simulink model "IEEE123bus_v2019b_Phasor_DPL_ZIPload"  (R2019b)
settings: Solver=VariableStepAuto  StartTime=0.0  StopTime=100  FixedStep=Ts  RelTol=1e-3
InitFcn:
  | a=1; % Loading Factor
  | Ts=0.1;% For Delay Blocks in Voltage Regulator Controls
  | 
  | % Simulation data for the IEEE 123 Node Test Feeder model
  | mi2km = 1.60934;%  miles to km conversion
  | ft2km = 0.0003048; % feet to km conversion
  | ms2F = 1*1e-6/(2*pi*60);% microsiemens to Farads conversion
  | 
  | %% Configuration 1
  | % Series Resitance and Reactance - ohm/mile
  | R_1 = [0.4576 0.1560 0.1535;0.1560 0.4666 0.1580;0.1535 0.1580 0.4615];
  | X_1 = [1.0780 0.5017 0.3849;0.5017 1.0482 0.4236;0.3849 0.4236 1.0651];
  | % charging susceptance - microsiemens/mile
  | B_1 = [5.6765 -1.8319 -0.6982;-1.8319 5.9809 -1.1645;-0.6982 -1.1645 5.3971];
  | 
  | R_1 = R_1/mi2km;
  | L_1 = (X_1/(2*pi*60))/mi2km;
  | C_1 =(B_1*ms2F)/mi2km;
  | 
  | %% Configuration 2 - series reactance - ohm/mile
  | R_2 = [0.4666 0.1580 0.1560;0.1580 0.4615 0.1535;0.1560 0.1535 0.4576];
  | X_2 = [1.0482 0.4236 0.5017;0.4236 1.0651 0.3849;0.5017 0.3849 1.0780];
  | % charging susceptance - microsiemens/mile
  | B_2 = [5.9809 -1.1645 -1.8319;-1.1645 5.3971 -0.6982;-1.8319 -0.6982 5.6765];
  | 
  | R_2 = R_2/mi2km;
  | L_2 = (X_2/(2*pi*60))/mi2km;
  | C_2 =(B_2*ms2F)/mi2km;
  | 
  | %% Configuration 3 - series reactance - ohm/mile
  | R_3 = [0.4615 0.1535 0.1580;0.1535 0.4576 0.1560;0.1580 0.1560 0.4666];
  | X_3 = [1.0651 0.3849 0.4236;0.3849 1.0780 0.5017;0.4236 0.5017 1.0482];
  | % charging susceptance - microsiemens/mile
  | B_3 = [5.3971 -0.6982 -1.1645;-0.6982 5.6765 -1.8319; -1.1645 -1.8319 5.9809];
  | 
  | R_3 = R_3/mi2km;
  | L_3 = (X_3/(2*pi*60))/mi2km;
  | C_3 =(B_3*ms2F)/mi2km;
  | 
  | %% Configuration 4 - series reactance - ohm/mile
  | R_4 = [0.4615 0.1580 0.1535;0.1580 0.4666 0.1560;0.1535 0.1560 0.4576];
  | X_4 = [1.0651 0.4236 0.3849;0.4236 1.0482 0.5017;0.3849 0.5017 1.0780];
  | % charging susceptance - microsiemens/mile
  | B_4 = [5.3971 -1.1645 -0.6982;-1.1645 5.9809 -1.8319;-0.6982 -1.8319 5.6765];
  | 
  | R_4 = R_4/mi2km;
  | L_4 = (X_4/(2*pi*60))/mi2km;
  | C_4 =(B_4*ms2F)/mi2km;
  | 
  | %% Configuration 5 - series reactance - ohm/mile
  | R_5 = [0.4666 0.1560 0.1580;0.1560 0.4576 0.1535;0.1580 0.1535 0.4615];
  | X_5 = [1.0482 0.5017 0.4236;0.5017 1.0780 0.3849;0.4236 0.3849 1.0651];
  | % charging susceptance - microsiemens/mile
  | B_5 = [5.9809 -1.8319 -1.1645;-1.8319 5.6765 -0.6982;-1.1645 -0.6982 5.3971];
  | 
  | R_5 = R_5/mi2km;
  | L_5 = (X_5/(2*pi*60))/mi2km;
  | C_5 =(B_5*ms2F)/mi2km;
  | 
  | %% Configuration 6 - series reactance - ohm/mile
  | ... (+68 lines)
undefined symbols (not defined in the file or in its folder): D1, Delta, find_system, j
libraries: powerlib x886, powerlib_meascontrol x31
(part 12 of 12)

== matlab function IEEE123bus_v2019b_Phasor_DPL_ZIPload/114 Y PQ/Embedded MATLAB Function ==
  data: Iinj output; Vmeas input; LoadType parameter; Vnom parameter; Pnom parameter; Qnom parameter; Vlim parameter
%Single Phase ZIP Load
%Author: Arun Suresh, University of North Carolina, Charlotte
%Iinj=((Pnom+jQnom)/Vmeas)'
function Iinj = InjectedCurrent(Vmeas,LoadType,Vnom,Pnom,Qnom,Vlim)
% Calculate Pl and Ql.
Kz=0;Ki=0;Kp=0;
Vk=(abs(Vmeas)/Vnom);%(Vmeas/Vnom)
switch LoadType  % 1 for Constant Z, 2 for Constant I and 3 for Constant P, 
    case 1
        Kz=1;
    case 2
        if Vk >= Vlim % convert to Constant Z load due to voltage violation
            Ki=1;
        else
            Kz=1;
        end
    case 3
        if Vk >= Vlim % convert to Constant Z load due to voltage violation
           Kp=1;
        else
            Kz=1;
        end          
 
end
Pl=Pnom *((Kz*Vk*Vk)+(Ki*Vk)+(Kp));
Ql=Qnom *((Kz*Vk*Vk)+(Ki*Vk)+(Kp));
% Net Injected Curent.
% j=sqrt(-1);
Iinj = conj((Pl+j*Ql)/Vmeas);

== matlab function IEEE123bus_v2019b_Phasor_DPL_ZIPload/113 Y Z/Embedded MATLAB Function ==
  data: Iinj output; Vmeas input; LoadType parameter; Vnom parameter; Pnom parameter; Qnom parameter; Vlim parameter
%Single Phase ZIP Load
%Author: Arun Suresh, University of North Carolina, Charlotte
%Iinj=((Pnom+jQnom)/Vmeas)'
function Iinj = InjectedCurrent(Vmeas,LoadType,Vnom,Pnom,Qnom,Vlim)
% Calculate Pl and Ql.
Kz=0;Ki=0;Kp=0;
Vk=(abs(Vmeas)/Vnom);%(Vmeas/Vnom)
switch LoadType  % 1 for Constant Z, 2 for Constant I and 3 for Constant P, 
    case 1
        Kz=1;
    case 2
        if Vk >= Vlim % convert to Constant Z load due to voltage violation
            Ki=1;
        else
            Kz=1;
        end
    case 3
        if Vk >= Vlim % convert to Constant Z load due to voltage violation
           Kp=1;
        else
            Kz=1;
        end          
 
end
Pl=Pnom *((Kz*Vk*Vk)+(Ki*Vk)+(Kp));
Ql=Qnom *((Kz*Vk*Vk)+(Ki*Vk)+(Kp));
% Net Injected Curent.
% j=sqrt(-1);
Iinj = conj((Pl+j*Ql)/Vmeas);

== matlab function IEEE123bus_v2019b_Phasor_DPL_ZIPload/112 Y I/Embedded MATLAB Function ==
  data: Iinj output; Vmeas input; LoadType parameter; Vnom parameter; Pnom parameter; Qnom parameter; Vlim parameter
%Single Phase ZIP Load
%Author: Arun Suresh, University of North Carolina, Charlotte
%Iinj=((Pnom+jQnom)/Vmeas)'
function Iinj = InjectedCurrent(Vmeas,LoadType,Vnom,Pnom,Qnom,Vlim)
% Calculate Pl and Ql.
Kz=0;Ki=0;Kp=0;
Vk=(abs(Vmeas)/Vnom);%(Vmeas/Vnom)
switch LoadType  % 1 for Constant Z, 2 for Constant I and 3 for Constant P, 
    case 1
        Kz=1;
    case 2
        if Vk >= Vlim % convert to Constant Z load due to voltage violation
            Ki=1;
        else
            Kz=1;
        end
    case 3
        if Vk >= Vlim % convert to Constant Z load due to voltage violation
           Kp=1;
        else
            Kz=1;
        end          
 
end
Pl=Pnom *((Kz*Vk*Vk)+(Ki*Vk)+(Kp));
Ql=Qnom *((Kz*Vk*Vk)+(Ki*Vk)+(Kp));
% Net Injected Curent.
% j=sqrt(-1);
Iinj = conj((Pl+j*Ql)/Vmeas);

== matlab function IEEE123bus_v2019b_Phasor_DPL_ZIPload/106 Y PQ/Embedded MATLAB Function ==
  data: Iinj output; Vmeas input; LoadType parameter; Vnom parameter; Pnom parameter; Qnom parameter; Vlim parameter
%Single Phase ZIP Load
%Author: Arun Suresh, University of North Carolina, Charlotte
%Iinj=((Pnom+jQnom)/Vmeas)'
function Iinj = InjectedCurrent(Vmeas,LoadType,Vnom,Pnom,Qnom,Vlim)
% Calculate Pl and Ql.
Kz=0;Ki=0;Kp=0;
Vk=(abs(Vmeas)/Vnom);%(Vmeas/Vnom)
switch LoadType  % 1 for Constant Z, 2 for Constant I and 3 for Constant P, 
    case 1
        Kz=1;
    case 2
        if Vk >= Vlim % convert to Constant Z load due to voltage violation
            Ki=1;
        else
            Kz=1;
        end
    case 3
        if Vk >= Vlim % convert to Constant Z load due to voltage violation
           Kp=1;
        else
            Kz=1;
        end          
 
end
Pl=Pnom *((Kz*Vk*Vk)+(Ki*Vk)+(Kp));
Ql=Qnom *((Kz*Vk*Vk)+(Ki*Vk)+(Kp));
% Net Injected Curent.
% j=sqrt(-1);
Iinj = conj((Pl+j*Ql)/Vmeas);

== matlab function IEEE123bus_v2019b_Phasor_DPL_ZIPload/107 Y PQ/Embedded MATLAB Function ==
  data: Iinj output; Vmeas input; LoadType parameter; Vnom parameter; Pnom parameter; Qnom parameter; Vlim parameter
%Single Phase ZIP Load
%Author: Arun Suresh, University of North Carolina, Charlotte
%Iinj=((Pnom+jQnom)/Vmeas)'
function Iinj = InjectedCurrent(Vmeas,LoadType,Vnom,Pnom,Qnom,Vlim)
% Calculate Pl and Ql.
Kz=0;Ki=0;Kp=0;
Vk=(abs(Vmeas)/Vnom);%(Vmeas/Vnom)
switch LoadType  % 1 for Constant Z, 2 for Constant I and 3 for Constant P, 
    case 1
        Kz=1;
    case 2
        if Vk >= Vlim % convert to Constant Z load due to voltage violation
            Ki=1;
        else
            Kz=1;
        end
    case 3
        if Vk >= Vlim % convert to Constant Z load due to voltage violation
           Kp=1;
        else
            Kz=1;
        end          
 
end
Pl=Pnom *((Kz*Vk*Vk)+(Ki*Vk)+(Kp));
Ql=Qnom *((Kz*Vk*Vk)+(Ki*Vk)+(Kp));
% Net Injected Curent.
% j=sqrt(-1);
Iinj = conj((Pl+j*Ql)/Vmeas);

== matlab function IEEE123bus_v2019b_Phasor_DPL_ZIPload/103 Y PQ/Embedded MATLAB Function ==
  data: Iinj output; Vmeas input; LoadType parameter; Vnom parameter; Pnom parameter; Qnom parameter; Vlim parameter
%Single Phase ZIP Load
%Author: Arun Suresh, University of North Carolina, Charlotte
%Iinj=((Pnom+jQnom)/Vmeas)'
function Iinj = InjectedCurrent(Vmeas,LoadType,Vnom,Pnom,Qnom,Vlim)
% Calculate Pl and Ql.
Kz=0;Ki=0;Kp=0;
Vk=(abs(Vmeas)/Vnom);%(Vmeas/Vnom)
switch LoadType  % 1 for Constant Z, 2 for Constant I and 3 for Constant P, 
    case 1
        Kz=1;
    case 2
        if Vk >= Vlim % convert to Constant Z load due to voltage violation
            Ki=1;
        else
            Kz=1;
        end
    case 3
        if Vk >= Vlim % convert to Constant Z load due to voltage violation
           Kp=1;
        else
            Kz=1;
        end          
 
end
Pl=Pnom *((Kz*Vk*Vk)+(Ki*Vk)+(Kp));
Ql=Qnom *((Kz*Vk*Vk)+(Ki*Vk)+(Kp));
% Net Injected Curent.
% j=sqrt(-1);
Iinj = conj((Pl+j*Ql)/Vmeas);

== matlab function IEEE123bus_v2019b_Phasor_DPL_ZIPload/104 Y PQ/Embedded MATLAB Function ==
  data: Iinj output; Vmeas input; LoadType parameter; Vnom parameter; Pnom parameter; Qnom parameter; Vlim parameter
%Single Phase ZIP Load
%Author: Arun Suresh, University of North Carolina, Charlotte
%Iinj=((Pnom+jQnom)/Vmeas)'
function Iinj = InjectedCurrent(Vmeas,LoadType,Vnom,Pnom,Qnom,Vlim)
% Calculate Pl and Ql.
Kz=0;Ki=0;Kp=0;
Vk=(abs(Vmeas)/Vnom);%(Vmeas/Vnom)
switch LoadType  % 1 for Constant Z, 2 for Constant I and 3 for Constant P, 
    case 1
        Kz=1;
    case 2
        if Vk >= Vlim % convert to Constant Z load due to voltage violation
            Ki=1;
        else
            Kz=1;
        end
    case 3
        if Vk >= Vlim % convert to Constant Z load due to voltage violation
           Kp=1;
        else
            Kz=1;
        end          
 
end
Pl=Pnom *((Kz*Vk*Vk)+(Ki*Vk)+(Kp));
Ql=Qnom *((Kz*Vk*Vk)+(Ki*Vk)+(Kp));
% Net Injected Curent.
% j=sqrt(-1);
Iinj = conj((Pl+j*Ql)/Vmeas);

== matlab function IEEE123bus_v2019b_Phasor_DPL_ZIPload/102 Y PQ/Embedded MATLAB Function ==
  data: Iinj output; Vmeas input; LoadType parameter; Vnom parameter; Pnom parameter; Qnom parameter; Vlim parameter
%Single Phase ZIP Load
%Author: Arun Suresh, University of North Carolina, Charlotte
%Iinj=((Pnom+jQnom)/Vmeas)'
function Iinj = InjectedCurrent(Vmeas,LoadType,Vnom,Pnom,Qnom,Vlim)
% Calculate Pl and Ql.
Kz=0;Ki=0;Kp=0;
Vk=(abs(Vmeas)/Vnom);%(Vmeas/Vnom)
switch LoadType  % 1 for Constant Z, 2 for Constant I and 3 for Constant P, 
    case 1
        Kz=1;
    case 2
        if Vk >= Vlim % convert to Constant Z load due to voltage violation
            Ki=1;
        else
            Kz=1;
        end
    case 3
        if Vk >= Vlim % convert to Constant Z load due to voltage violation
           Kp=1;
        else
            Kz=1;
        end          
 
end
Pl=Pnom *((Kz*Vk*Vk)+(Ki*Vk)+(Kp));
Ql=Qnom *((Kz*Vk*Vk)+(Ki*Vk)+(Kp));
% Net Injected Curent.
% j=sqrt(-1);
Iinj = conj((Pl+j*Ql)/Vmeas);

== matlab function IEEE123bus_v2019b_Phasor_DPL_ZIPload/98 Y PQ/Embedded MATLAB Function ==
  data: Iinj output; Vmeas input; LoadType parameter; Vnom parameter; Pnom parameter; Qnom parameter; Vlim parameter
%Single Phase ZIP Load
%Author: Arun Suresh, University of North Carolina, Charlotte
%Iinj=((Pnom+jQnom)/Vmeas)'
function Iinj = InjectedCurrent(Vmeas,LoadType,Vnom,Pnom,Qnom,Vlim)
% Calculate Pl and Ql.
Kz=0;Ki=0;Kp=0;
Vk=(abs(Vmeas)/Vnom);%(Vmeas/Vnom)
switch LoadType  % 1 for Constant Z, 2 for Constant I and 3 for Constant P, 
    case 1
        Kz=1;
    case 2
        if Vk >= Vlim % convert to Constant Z load due to voltage violation
            Ki=1;
        else
            Kz=1;
        end
    case 3
        if Vk >= Vlim % convert to Constant Z load due to voltage violation
           Kp=1;
        else
            Kz=1;
        end          
 
end
Pl=Pnom *((Kz*Vk*Vk)+(Ki*Vk)+(Kp));
Ql=Qnom *((Kz*Vk*Vk)+(Ki*Vk)+(Kp));
% Net Injected Curent.
% j=sqrt(-1);
Iinj = conj((Pl+j*Ql)/Vmeas);

== matlab function IEEE123bus_v2019b_Phasor_DPL_ZIPload/99 Y PQ/Embedded MATLAB Function ==
  data: Iinj output; Vmeas input; LoadType parameter; Vnom parameter; Pnom parameter; Qnom parameter; Vlim parameter
%Single Phase ZIP Load
%Author: Arun Suresh, University of North Carolina, Charlotte
%Iinj=((Pnom+jQnom)/Vmeas)'
function Iinj = InjectedCurrent(Vmeas,LoadType,Vnom,Pnom,Qnom,Vlim)
% Calculate Pl and Ql.
Kz=0;Ki=0;Kp=0;
Vk=(abs(Vmeas)/Vnom);%(Vmeas/Vnom)
switch LoadType  % 1 for Constant Z, 2 for Constant I and 3 for Constant P, 
    case 1
        Kz=1;
    case 2
        if Vk >= Vlim % convert to Constant Z load due to voltage violation
            Ki=1;
        else
            Kz=1;
        end
    case 3
        if Vk >= Vlim % convert to Constant Z load due to voltage violation
           Kp=1;
        else
            Kz=1;
        end          
 
end
Pl=Pnom *((Kz*Vk*Vk)+(Ki*Vk)+(Kp));
Ql=Qnom *((Kz*Vk*Vk)+(Ki*Vk)+(Kp));
% Net Injected Curent.
% j=sqrt(-1);
Iinj = conj((Pl+j*Ql)/Vmeas);

== matlab function IEEE123bus_v2019b_Phasor_DPL_ZIPload/100 Y Z/Embedded MATLAB Function ==
  data: Iinj output; Vmeas input; LoadType parameter; Vnom parameter; Pnom parameter; Qnom parameter; Vlim parameter
%Single Phase ZIP Load
%Author: Arun Suresh, University of North Carolina, Charlotte
%Iinj=((Pnom+jQnom)/Vmeas)'
function Iinj = InjectedCurrent(Vmeas,LoadType,Vnom,Pnom,Qnom,Vlim)
% Calculate Pl and Ql.
Kz=0;Ki=0;Kp=0;
Vk=(abs(Vmeas)/Vnom);%(Vmeas/Vnom)
switch LoadType  % 1 for Constant Z, 2 for Constant I and 3 for Constant P, 
    case 1
        Kz=1;
    case 2
        if Vk >= Vlim % convert to Constant Z load due to voltage violation
            Ki=1;
        else
            Kz=1;
        end
    case 3
        if Vk >= Vlim % convert to Constant Z load due to voltage violation
           Kp=1;
        else
            Kz=1;
        end          
 
end
Pl=Pnom *((Kz*Vk*Vk)+(Ki*Vk)+(Kp));
Ql=Qnom *((Kz*Vk*Vk)+(Ki*Vk)+(Kp));
% Net Injected Curent.
% j=sqrt(-1);
Iinj = conj((Pl+j*Ql)/Vmeas);

== matlab function IEEE123bus_v2019b_Phasor_DPL_ZIPload/71 Y PQ/Embedded MATLAB Function ==
  data: Iinj output; Vmeas input; LoadType parameter; Vnom parameter; Pnom parameter; Qnom parameter; Vlim parameter
%Single Phase ZIP Load
%Author: Arun Suresh, University of North Carolina, Charlotte
%Iinj=((Pnom+jQnom)/Vmeas)'
function Iinj = InjectedCurrent(Vmeas,LoadType,Vnom,Pnom,Qnom,Vlim)
% Calculate Pl and Ql.
Kz=0;Ki=0;Kp=0;
Vk=(abs(Vmeas)/Vnom);%(Vmeas/Vnom)
switch LoadType  % 1 for Constant Z, 2 for Constant I and 3 for Constant P, 
    case 1
        Kz=1;
    case 2
        if Vk >= Vlim % convert to Constant Z load due to voltage violation
            Ki=1;
        else
            Kz=1;
        end
    case 3
        if Vk >= Vlim % convert to Constant Z load due to voltage violation
           Kp=1;
        else
            Kz=1;
        end          
 
end
Pl=Pnom *((Kz*Vk*Vk)+(Ki*Vk)+(Kp));
Ql=Qnom *((Kz*Vk*Vk)+(Ki*Vk)+(Kp));
% Net Injected Curent.
% j=sqrt(-1);
Iinj = conj((Pl+j*Ql)/Vmeas);

== matlab function IEEE123bus_v2019b_Phasor_DPL_ZIPload/69 Y PQ/Embedded MATLAB Function ==
  data: Iinj output; Vmeas input; LoadType parameter; Vnom parameter; Pnom parameter; Qnom parameter; Vlim parameter
%Single Phase ZIP Load
%Author: Arun Suresh, University of North Carolina, Charlotte
%Iinj=((Pnom+jQnom)/Vmeas)'
function Iinj = InjectedCurrent(Vmeas,LoadType,Vnom,Pnom,Qnom,Vlim)
% Calculate Pl and Ql.
Kz=0;Ki=0;Kp=0;
Vk=(abs(Vmeas)/Vnom);%(Vmeas/Vnom)
switch LoadType  % 1 for Constant Z, 2 for Constant I and 3 for Constant P, 
    case 1
        Kz=1;
    case 2
        if Vk >= Vlim % convert to Constant Z load due to voltage violation
            Ki=1;
        else
            Kz=1;
        end
    case 3
        if Vk >= Vlim % convert to Constant Z load due to voltage violation
           Kp=1;
        else
            Kz=1;
        end          
 
end
Pl=Pnom *((Kz*Vk*Vk)+(Ki*Vk)+(Kp));
Ql=Qnom *((Kz*Vk*Vk)+(Ki*Vk)+(Kp));
% Net Injected Curent.
% j=sqrt(-1);
Iinj = conj((Pl+j*Ql)/Vmeas);

== matlab function IEEE123bus_v2019b_Phasor_DPL_ZIPload/68 Y PQ/Embedded MATLAB Function ==
  data: Iinj output; Vmeas input; LoadType parameter; Vnom parameter; Pnom parameter; Qnom parameter; Vlim parameter
%Single Phase ZIP Load
%Author: Arun Suresh, University of North Carolina, Charlotte
%Iinj=((Pnom+jQnom)/Vmeas)'
function Iinj = InjectedCurrent(Vmeas,LoadType,Vnom,Pnom,Qnom,Vlim)
% Calculate Pl and Ql.
Kz=0;Ki=0;Kp=0;
Vk=(abs(Vmeas)/Vnom);%(Vmeas/Vnom)
switch LoadType  % 1 for Constant Z, 2 for Constant I and 3 for Constant P, 
    case 1
        Kz=1;
    case 2
        if Vk >= Vlim % convert to Constant Z load due to voltage violation
            Ki=1;
        else
            Kz=1;
        end
    case 3
        if Vk >= Vlim % convert to Constant Z load due to voltage violation
           Kp=1;
        else
            Kz=1;
        end          
 
end
Pl=Pnom *((Kz*Vk*Vk)+(Ki*Vk)+(Kp));
Ql=Qnom *((Kz*Vk*Vk)+(Ki*Vk)+(Kp));
% Net Injected Curent.
% j=sqrt(-1);
Iinj = conj((Pl+j*Ql)/Vmeas);

== matlab function IEEE123bus_v2019b_Phasor_DPL_ZIPload/70 Y PQ/Embedded MATLAB Function ==
  data: Iinj output; Vmeas input; LoadType parameter; Vnom parameter; Pnom parameter; Qnom parameter; Vlim parameter
%Single Phase ZIP Load
%Author: Arun Suresh, University of North Carolina, Charlotte
%Iinj=((Pnom+jQnom)/Vmeas)'
function Iinj = InjectedCurrent(Vmeas,LoadType,Vnom,Pnom,Qnom,Vlim)
% Calculate Pl and Ql.
Kz=0;Ki=0;Kp=0;
Vk=(abs(Vmeas)/Vnom);%(Vmeas/Vnom)
switch LoadType  % 1 for Constant Z, 2 for Constant I and 3 for Constant P, 
    case 1
        Kz=1;
    case 2
        if Vk >= Vlim % convert to Constant Z load due to voltage violation
            Ki=1;
        else
            Kz=1;
        end
    case 3
        if Vk >= Vlim % convert to Constant Z load due to voltage violation
           Kp=1;
        else
            Kz=1;
        end          
 
end
Pl=Pnom *((Kz*Vk*Vk)+(Ki*Vk)+(Kp));
Ql=Qnom *((Kz*Vk*Vk)+(Ki*Vk)+(Kp));
% Net Injected Curent.
% j=sqrt(-1);
Iinj = conj((Pl+j*Ql)/Vmeas);

== matlab function IEEE123bus_v2019b_Phasor_DPL_ZIPload/73 Y PQ/Embedded MATLAB Function ==
  data: Iinj output; Vmeas input; LoadType parameter; Vnom parameter; Pnom parameter; Qnom parameter; Vlim parameter
%Single Phase ZIP Load
%Author: Arun Suresh, University of North Carolina, Charlotte
%Iinj=((Pnom+jQnom)/Vmeas)'
function Iinj = InjectedCurrent(Vmeas,LoadType,Vnom,Pnom,Qnom,Vlim)
% Calculate Pl and Ql.
Kz=0;Ki=0;Kp=0;
Vk=(abs(Vmeas)/Vnom);%(Vmeas/Vnom)
switch LoadType  % 1 for Constant Z, 2 for Constant I and 3 for Constant P, 
    case 1
        Kz=1;
    case 2
        if Vk >= Vlim % convert to Constant Z load due to voltage violation
            Ki=1;
        else
            Kz=1;
        end
    case 3
        if Vk >= Vlim % convert to Constant Z load due to voltage violation
           Kp=1;
        else
            Kz=1;
        end          
 
end
Pl=Pnom *((Kz*Vk*Vk)+(Ki*Vk)+(Kp));
Ql=Qnom *((Kz*Vk*Vk)+(Ki*Vk)+(Kp));
% Net Injected Curent.
% j=sqrt(-1);
Iinj = conj((Pl+j*Ql)/Vmeas);

== matlab function IEEE123bus_v2019b_Phasor_DPL_ZIPload/75 Y PQ/Embedded MATLAB Function ==
  data: Iinj output; Vmeas input; LoadType parameter; Vnom parameter; Pnom parameter; Qnom parameter; Vlim parameter
%Single Phase ZIP Load
%Author: Arun Suresh, University of North Carolina, Charlotte
%Iinj=((Pnom+jQnom)/Vmeas)'
function Iinj = InjectedCurrent(Vmeas,LoadType,Vnom,Pnom,Qnom,Vlim)
% Calculate Pl and Ql.
Kz=0;Ki=0;Kp=0;
Vk=(abs(Vmeas)/Vnom);%(Vmeas/Vnom)
switch LoadType  % 1 for Constant Z, 2 for Constant I and 3 for Constant P, 
    case 1
        Kz=1;
    case 2
        if Vk >= Vlim % convert to Constant Z load due to voltage violation
            Ki=1;
        else
            Kz=1;
        end
    case 3
        if Vk >= Vlim % convert to Constant Z load due to voltage violation
           Kp=1;
        else
            Kz=1;
        end          
 
end
Pl=Pnom *((Kz*Vk*Vk)+(Ki*Vk)+(Kp));
Ql=Qnom *((Kz*Vk*Vk)+(Ki*Vk)+(Kp));
% Net Injected Curent.
% j=sqrt(-1);
Iinj = conj((Pl+j*Ql)/Vmeas);

== matlab function IEEE123bus_v2019b_Phasor_DPL_ZIPload/74 Y Z/Embedded MATLAB Function ==
  data: Iinj output; Vmeas input; LoadType parameter; Vnom parameter; Pnom parameter; Qnom parameter; Vlim parameter
%Single Phase ZIP Load
%Author: Arun Suresh, University of North Carolina, Charlotte
%Iinj=((Pnom+jQnom)/Vmeas)'
function Iinj = InjectedCurrent(Vmeas,LoadType,Vnom,Pnom,Qnom,Vlim)
% Calculate Pl and Ql.
Kz=0;Ki=0;Kp=0;
Vk=(abs(Vmeas)/Vnom);%(Vmeas/Vnom)
switch LoadType  % 1 for Constant Z, 2 for Constant I and 3 for Constant P, 
    case 1
        Kz=1;
    case 2
        if Vk >= Vlim % convert to Constant Z load due to voltage violation
            Ki=1;
        else
            Kz=1;
        end
    case 3
        if Vk >= Vlim % convert to Constant Z load due to voltage violation
           Kp=1;
        else
            Kz=1;
        end          
 
end
Pl=Pnom *((Kz*Vk*Vk)+(Ki*Vk)+(Kp));
Ql=Qnom *((Kz*Vk*Vk)+(Ki*Vk)+(Kp));
% Net Injected Curent.
% j=sqrt(-1);
Iinj = conj((Pl+j*Ql)/Vmeas);

== matlab function IEEE123bus_v2019b_Phasor_DPL_ZIPload/77 Y PQ/Embedded MATLAB Function ==
  data: Iinj output; Vmeas input; LoadType parameter; Vnom parameter; Pnom parameter; Qnom parameter; Vlim parameter
%Single Phase ZIP Load
%Author: Arun Suresh, University of North Carolina, Charlotte
%Iinj=((Pnom+jQnom)/Vmeas)'
function Iinj = InjectedCurrent(Vmeas,LoadType,Vnom,Pnom,Qnom,Vlim)
% Calculate Pl and Ql.
Kz=0;Ki=0;Kp=0;
Vk=(abs(Vmeas)/Vnom);%(Vmeas/Vnom)
switch LoadType  % 1 for Constant Z, 2 for Constant I and 3 for Constant P, 
    case 1
        Kz=1;
    case 2
        if Vk >= Vlim % convert to Constant Z load due to voltage violation
            Ki=1;
        else
            Kz=1;
        end
    case 3
        if Vk >= Vlim % convert to Constant Z load due to voltage violation
           Kp=1;
        else
            Kz=1;
        end          
 
end
Pl=Pnom *((Kz*Vk*Vk)+(Ki*Vk)+(Kp));
Ql=Qnom *((Kz*Vk*Vk)+(Ki*Vk)+(Kp));
% Net Injected Curent.
% j=sqrt(-1);
Iinj = conj((Pl+j*Ql)/Vmeas);

== matlab function IEEE123bus_v2019b_Phasor_DPL_ZIPload/79 Y Z/Embedded MATLAB Function ==
  data: Iinj output; Vmeas input; LoadType parameter; Vnom parameter; Pnom parameter; Qnom parameter; Vlim parameter
%Single Phase ZIP Load
%Author: Arun Suresh, University of North Carolina, Charlotte
%Iinj=((Pnom+jQnom)/Vmeas)'
function Iinj = InjectedCurrent(Vmeas,LoadType,Vnom,Pnom,Qnom,Vlim)
% Calculate Pl and Ql.
Kz=0;Ki=0;Kp=0;
Vk=(abs(Vmeas)/Vnom);%(Vmeas/Vnom)
switch LoadType  % 1 for Constant Z, 2 for Constant I and 3 for Constant P, 
    case 1
        Kz=1;
    case 2
        if Vk >= Vlim % convert to Constant Z load due to voltage violation
            Ki=1;
        else
            Kz=1;
        end
    case 3
        if Vk >= Vlim % convert to Constant Z load due to voltage violation
           Kp=1;
        else
            Kz=1;
        end          
 
end
Pl=Pnom *((Kz*Vk*Vk)+(Ki*Vk)+(Kp));
Ql=Qnom *((Kz*Vk*Vk)+(Ki*Vk)+(Kp));
% Net Injected Curent.
% j=sqrt(-1);
Iinj = conj((Pl+j*Ql)/Vmeas);

== matlab function IEEE123bus_v2019b_Phasor_DPL_ZIPload/80 Y PQ/Embedded MATLAB Function ==
  data: Iinj output; Vmeas input; LoadType parameter; Vnom parameter; Pnom parameter; Qnom parameter; Vlim parameter
%Single Phase ZIP Load
%Author: Arun Suresh, University of North Carolina, Charlotte
%Iinj=((Pnom+jQnom)/Vmeas)'
function Iinj = InjectedCurrent(Vmeas,LoadType,Vnom,Pnom,Qnom,Vlim)
% Calculate Pl and Ql.
Kz=0;Ki=0;Kp=0;
Vk=(abs(Vmeas)/Vnom);%(Vmeas/Vnom)
switch LoadType  % 1 for Constant Z, 2 for Constant I and 3 for Constant P, 
    case 1
        Kz=1;
    case 2
        if Vk >= Vlim % convert to Constant Z load due to voltage violation
            Ki=1;
        else
            Kz=1;
        end
    case 3
        if Vk >= Vlim % convert to Constant Z load due to voltage violation
           Kp=1;
        else
            Kz=1;
        end          
 
end
Pl=Pnom *((Kz*Vk*Vk)+(Ki*Vk)+(Kp));
Ql=Qnom *((Kz*Vk*Vk)+(Ki*Vk)+(Kp));
% Net Injected Curent.
% j=sqrt(-1);
Iinj = conj((Pl+j*Ql)/Vmeas);

== matlab function IEEE123bus_v2019b_Phasor_DPL_ZIPload/84 Y PQ/Embedded MATLAB Function ==
  data: Iinj output; Vmeas input; LoadType parameter; Vnom parameter; Pnom parameter; Qnom parameter; Vlim parameter
%Single Phase ZIP Load
%Author: Arun Suresh, University of North Carolina, Charlotte
%Iinj=((Pnom+jQnom)/Vmeas)'
function Iinj = InjectedCurrent(Vmeas,LoadType,Vnom,Pnom,Qnom,Vlim)
% Calculate Pl and Ql.
Kz=0;Ki=0;Kp=0;
Vk=(abs(Vmeas)/Vnom);%(Vmeas/Vnom)
switch LoadType  % 1 for Constant Z, 2 for Constant I and 3 for Constant P, 
    case 1
        Kz=1;
    case 2
        if Vk >= Vlim % convert to Constant Z load due to voltage violation
            Ki=1;
        else
            Kz=1;
        end
    case 3
        if Vk >= Vlim % convert to Constant Z load due to voltage violation
           Kp=1;
        else
            Kz=1;
        end          
 
end
Pl=Pnom *((Kz*Vk*Vk)+(Ki*Vk)+(Kp));
Ql=Qnom *((Kz*Vk*Vk)+(Ki*Vk)+(Kp));
% Net Injected Curent.
% j=sqrt(-1);
Iinj = conj((Pl+j*Ql)/Vmeas);

== matlab function IEEE123bus_v2019b_Phasor_DPL_ZIPload/85 Y PQ/Embedded MATLAB Function ==
  data: Iinj output; Vmeas input; LoadType parameter; Vnom parameter; Pnom parameter; Qnom parameter; Vlim parameter
%Single Phase ZIP Load
%Author: Arun Suresh, University of North Carolina, Charlotte
%Iinj=((Pnom+jQnom)/Vmeas)'
function Iinj = InjectedCurrent(Vmeas,LoadType,Vnom,Pnom,Qnom,Vlim)
% Calculate Pl and Ql.
Kz=0;Ki=0;Kp=0;
Vk=(abs(Vmeas)/Vnom);%(Vmeas/Vnom)
switch LoadType  % 1 for Constant Z, 2 for Constant I and 3 for Constant P, 
    case 1
        Kz=1;
    case 2
        if Vk >= Vlim % convert to Constant Z load due to voltage violation
            Ki=1;
        else
            Kz=1;
        end
    case 3
        if Vk >= Vlim % convert to Constant Z load due to voltage violation
           Kp=1;
        else
            Kz=1;
        end          
 
end
Pl=Pnom *((Kz*Vk*Vk)+(Ki*Vk)+(Kp));
Ql=Qnom *((Kz*Vk*Vk)+(Ki*Vk)+(Kp));
% Net Injected Curent.
% j=sqrt(-1);
Iinj = conj((Pl+j*Ql)/Vmeas);

== matlab function IEEE123bus_v2019b_Phasor_DPL_ZIPload/83 Y PQ/Embedded MATLAB Function ==
  data: Iinj output; Vmeas input; LoadType parameter; Vnom parameter; Pnom parameter; Qnom parameter; Vlim parameter
%Single Phase ZIP Load
%Author: Arun Suresh, University of North Carolina, Charlotte
%Iinj=((Pnom+jQnom)/Vmeas)'
function Iinj = InjectedCurrent(Vmeas,LoadType,Vnom,Pnom,Qnom,Vlim)
% Calculate Pl and Ql.
Kz=0;Ki=0;Kp=0;
Vk=(abs(Vmeas)/Vnom);%(Vmeas/Vnom)
switch LoadType  % 1 for Constant Z, 2 for Constant I and 3 for Constant P, 
    case 1
        Kz=1;
    case 2
        if Vk >= Vlim % convert to Constant Z load due to voltage violation
            Ki=1;
        else
            Kz=1;
        end
    case 3
        if Vk >= Vlim % convert to Constant Z load due to voltage violation
           Kp=1;
        else
            Kz=1;
        end          
 
end
Pl=Pnom *((Kz*Vk*Vk)+(Ki*Vk)+(Kp));
Ql=Qnom *((Kz*Vk*Vk)+(Ki*Vk)+(Kp));
% Net Injected Curent.
% j=sqrt(-1);
Iinj = conj((Pl+j*Ql)/Vmeas);

== matlab function IEEE123bus_v2019b_Phasor_DPL_ZIPload/82 Y PQ/Embedded MATLAB Function ==
  data: Iinj output; Vmeas input; LoadType parameter; Vnom parameter; Pnom parameter; Qnom parameter; Vlim parameter
%Single Phase ZIP Load
%Author: Arun Suresh, University of North Carolina, Charlotte
%Iinj=((Pnom+jQnom)/Vmeas)'
function Iinj = InjectedCurrent(Vmeas,LoadType,Vnom,Pnom,Qnom,Vlim)
% Calculate Pl and Ql.
Kz=0;Ki=0;Kp=0;
Vk=(abs(Vmeas)/Vnom);%(Vmeas/Vnom)
switch LoadType  % 1 for Constant Z, 2 for Constant I and 3 for Constant P, 
    case 1
        Kz=1;
    case 2
        if Vk >= Vlim % convert to Constant Z load due to voltage violation
            Ki=1;
        else
            Kz=1;
        end
    case 3
        if Vk >= Vlim % convert to Constant Z load due to voltage violation
           Kp=1;
        else
            Kz=1;
        end          
 
end
Pl=Pnom *((Kz*Vk*Vk)+(Ki*Vk)+(Kp));
Ql=Qnom *((Kz*Vk*Vk)+(Ki*Vk)+(Kp));
% Net Injected Curent.
% j=sqrt(-1);
Iinj = conj((Pl+j*Ql)/Vmeas);

== matlab function IEEE123bus_v2019b_Phasor_DPL_ZIPload/86 Y PQ/Embedded MATLAB Function ==
  data: Iinj output; Vmeas input; LoadType parameter; Vnom parameter; Pnom parameter; Qnom parameter; Vlim parameter
%Single Phase ZIP Load
%Author: Arun Suresh, University of North Carolina, Charlotte
%Iinj=((Pnom+jQnom)/Vmeas)'
function Iinj = InjectedCurrent(Vmeas,LoadType,Vnom,Pnom,Qnom,Vlim)
% Calculate Pl and Ql.
Kz=0;Ki=0;Kp=0;
Vk=(abs(Vmeas)/Vnom);%(Vmeas/Vnom)
switch LoadType  % 1 for Constant Z, 2 for Constant I and 3 for Constant P, 
    case 1
        Kz=1;
    case 2
        if Vk >= Vlim % convert to Constant Z load due to voltage violation
            Ki=1;
        else
            Kz=1;
        end
    case 3
        if Vk >= Vlim % convert to Constant Z load due to voltage violation
           Kp=1;
        else
            Kz=1;
        end          
 
end
Pl=Pnom *((Kz*Vk*Vk)+(Ki*Vk)+(Kp));
Ql=Qnom *((Kz*Vk*Vk)+(Ki*Vk)+(Kp));
% Net Injected Curent.
% j=sqrt(-1);
Iinj = conj((Pl+j*Ql)/Vmeas);

== matlab function IEEE123bus_v2019b_Phasor_DPL_ZIPload/76 DI/Embedded MATLAB Function2 ==
  data: Iinj output; Vmeas input; LoadType parameter; Vnom parameter; Pnom parameter; Qnom parameter; Vlim parameter
%Three Phase Delta ZIP Load
%Author: Arun Suresh, University of North Carolina, Charlotte
%Pl=Pnom(Kz*(Vmeas/Vnom)^2+Ki(Vmeas/Vnom)+Kp), nom-nominal value,meas-measured value
%Ql=Qnom(Kz*(Vmeas/Vnom)^2+Ki(Vmeas/Vnom)+Kp), nom-nominal value,meas-measured value
%Iinj=((Pl+jQl)/Vmeas)'
function Iinj = InjectedCurrent(Vmeas,LoadType,Vnom,Pnom,Qnom,Vlim)
% % Calculate Pl and Ql.
Kz=0;Ki=0;Kp=0;
Vk=(abs(Vmeas)/(Vnom));%(Vmeas/Vnom)
switch LoadType  % 1 for Constant Z, 2 for Constant I and 3 for Constant P, 
    case 1
        Kz=1;
    case 2
        if Vk >= Vlim % convert to Constant Z load due to voltage violation
            Ki=1;
        else
            Kz=1;
        end
    case 3
        if Vk >= Vlim % convert to Constant Z load due to voltage violation
           Kp=1;
        else
            Kz=1;
        end          
 
end
Pl=Pnom'.*((Kz*Vk.*Vk)+(Ki*Vk)+(Kp));
Ql=Qnom'.*((Kz*Vk.*Vk)+(Ki*Vk)+(Kp));
% Net Injected Curent.
% j=sqrt(-1);
Iinj = conj((Pl+j*Ql)./Vmeas);

== matlab function IEEE123bus_v2019b_Phasor_DPL_ZIPload/88 Y PQ/Embedded MATLAB Function ==
  data: Iinj output; Vmeas input; LoadType parameter; Vnom parameter; Pnom parameter; Qnom parameter; Vlim parameter
%Single Phase ZIP Load
%Author: Arun Suresh, University of North Carolina, Charlotte
%Iinj=((Pnom+jQnom)/Vmeas)'
function Iinj = InjectedCurrent(Vmeas,LoadType,Vnom,Pnom,Qnom,Vlim)
% Calculate Pl and Ql.
Kz=0;Ki=0;Kp=0;
Vk=(abs(Vmeas)/Vnom);%(Vmeas/Vnom)
switch LoadType  % 1 for Constant Z, 2 for Constant I and 3 for Constant P, 
    case 1
        Kz=1;
    case 2
        if Vk >= Vlim % convert to Constant Z load due to voltage violation
            Ki=1;
        else
            Kz=1;
        end
    case 3
        if Vk >= Vlim % convert to Constant Z load due to voltage violation
           Kp=1;
        else
            Kz=1;
        end          
 
end
Pl=Pnom *((Kz*Vk*Vk)+(Ki*Vk)+(Kp));
Ql=Qnom *((Kz*Vk*Vk)+(Ki*Vk)+(Kp));
% Net Injected Curent.
% j=sqrt(-1);
Iinj = conj((Pl+j*Ql)/Vmeas);

== matlab function IEEE123bus_v2019b_Phasor_DPL_ZIPload/87 Y PQ/Embedded MATLAB Function ==
  data: Iinj output; Vmeas input; LoadType parameter; Vnom parameter; Pnom parameter; Qnom parameter; Vlim parameter
%Single Phase ZIP Load
%Author: Arun Suresh, University of North Carolina, Charlotte
%Iinj=((Pnom+jQnom)/Vmeas)'
function Iinj = InjectedCurrent(Vmeas,LoadType,Vnom,Pnom,Qnom,Vlim)
% Calculate Pl and Ql.
Kz=0;Ki=0;Kp=0;
Vk=(abs(Vmeas)/Vnom);%(Vmeas/Vnom)
switch LoadType  % 1 for Constant Z, 2 for Constant I and 3 for Constant P, 
    case 1
        Kz=1;
    case 2
        if Vk >= Vlim % convert to Constant Z load due to voltage violation
            Ki=1;
        else
            Kz=1;
        end
    case 3
        if Vk >= Vlim % convert to Constant Z load due to voltage violation
           Kp=1;
        else
            Kz=1;
        end          
 
end
Pl=Pnom *((Kz*Vk*Vk)+(Ki*Vk)+(Kp));
Ql=Qnom *((Kz*Vk*Vk)+(Ki*Vk)+(Kp));
% Net Injected Curent.
% j=sqrt(-1);
Iinj = conj((Pl+j*Ql)/Vmeas);

== matlab function IEEE123bus_v2019b_Phasor_DPL_ZIPload/90 Y I/Embedded MATLAB Function ==
  data: Iinj output; Vmeas input; LoadType parameter; Vnom parameter; Pnom parameter; Qnom parameter; Vlim parameter
%Single Phase ZIP Load
%Author: Arun Suresh, University of North Carolina, Charlotte
%Iinj=((Pnom+jQnom)/Vmeas)'
function Iinj = InjectedCurrent(Vmeas,LoadType,Vnom,Pnom,Qnom,Vlim)
% Calculate Pl and Ql.
Kz=0;Ki=0;Kp=0;
Vk=(abs(Vmeas)/Vnom);%(Vmeas/Vnom)
switch LoadType  % 1 for Constant Z, 2 for Constant I and 3 for Constant P, 
    case 1
        Kz=1;
    case 2
        if Vk >= Vlim % convert to Constant Z load due to voltage violation
            Ki=1;
        else
            Kz=1;
        end
    case 3
        if Vk >= Vlim % convert to Constant Z load due to voltage violation
           Kp=1;
        else
            Kz=1;
        end          
 
end
Pl=Pnom *((Kz*Vk*Vk)+(Ki*Vk)+(Kp));
Ql=Qnom *((Kz*Vk*Vk)+(Ki*Vk)+(Kp));
% Net Injected Curent.
% j=sqrt(-1);
Iinj = conj((Pl+j*Ql)/Vmeas);

== matlab function IEEE123bus_v2019b_Phasor_DPL_ZIPload/92 Y PQ/Embedded MATLAB Function ==
  data: Iinj output; Vmeas input; LoadType parameter; Vnom parameter; Pnom parameter; Qnom parameter; Vlim parameter
%Single Phase ZIP Load
%Author: Arun Suresh, University of North Carolina, Charlotte
%Iinj=((Pnom+jQnom)/Vmeas)'
function Iinj = InjectedCurrent(Vmeas,LoadType,Vnom,Pnom,Qnom,Vlim)
% Calculate Pl and Ql.
Kz=0;Ki=0;Kp=0;
Vk=(abs(Vmeas)/Vnom);%(Vmeas/Vnom)
switch LoadType  % 1 for Constant Z, 2 for Constant I and 3 for Constant P, 
    case 1
        Kz=1;
    case 2
        if Vk >= Vlim % convert to Constant Z load due to voltage violation
            Ki=1;
        else
            Kz=1;
        end
    case 3
        if Vk >= Vlim % convert to Constant Z load due to voltage violation
           Kp=1;
        else
            Kz=1;
        end          
 
end
Pl=Pnom *((Kz*Vk*Vk)+(Ki*Vk)+(Kp));
Ql=Qnom *((Kz*Vk*Vk)+(Ki*Vk)+(Kp));
% Net Injected Curent.
% j=sqrt(-1);
Iinj = conj((Pl+j*Ql)/Vmeas);

== matlab function IEEE123bus_v2019b_Phasor_DPL_ZIPload/94 Y PQ/Embedded MATLAB Function ==
  data: Iinj output; Vmeas input; LoadType parameter; Vnom parameter; Pnom parameter; Qnom parameter; Vlim parameter
%Single Phase ZIP Load
%Author: Arun Suresh, University of North Carolina, Charlotte
%Iinj=((Pnom+jQnom)/Vmeas)'
function Iinj = InjectedCurrent(Vmeas,LoadType,Vnom,Pnom,Qnom,Vlim)
% Calculate Pl and Ql.
Kz=0;Ki=0;Kp=0;
Vk=(abs(Vmeas)/Vnom);%(Vmeas/Vnom)
switch LoadType  % 1 for Constant Z, 2 for Constant I and 3 for Constant P, 
    case 1
        Kz=1;
    case 2
        if Vk >= Vlim % convert to Constant Z load due to voltage violation
            Ki=1;
        else
            Kz=1;
        end
    case 3
        if Vk >= Vlim % convert to Constant Z load due to voltage violation
           Kp=1;
        else
            Kz=1;
        end          
 
end
Pl=Pnom *((Kz*Vk*Vk)+(Ki*Vk)+(Kp));
Ql=Qnom *((Kz*Vk*Vk)+(Ki*Vk)+(Kp));
% Net Injected Curent.
% j=sqrt(-1);
Iinj = conj((Pl+j*Ql)/Vmeas);

== matlab function IEEE123bus_v2019b_Phasor_DPL_ZIPload/96 Y PQ/Embedded MATLAB Function ==
  data: Iinj output; Vmeas input; LoadType parameter; Vnom parameter; Pnom parameter; Qnom parameter; Vlim parameter
%Single Phase ZIP Load
%Author: Arun Suresh, University of North Carolina, Charlotte
%Iinj=((Pnom+jQnom)/Vmeas)'
function Iinj = InjectedCurrent(Vmeas,LoadType,Vnom,Pnom,Qnom,Vlim)
% Calculate Pl and Ql.
Kz=0;Ki=0;Kp=0;
Vk=(abs(Vmeas)/Vnom);%(Vmeas/Vnom)
switch LoadType  % 1 for Constant Z, 2 for Constant I and 3 for Constant P, 
    case 1
        Kz=1;
    case 2
        if Vk >= Vlim % convert to Constant Z load due to voltage violation
            Ki=1;
        else
            Kz=1;
        end
    case 3
        if Vk >= Vlim % convert to Constant Z load due to voltage violation
           Kp=1;
        else
            Kz=1;
        end          
 
end
Pl=Pnom *((Kz*Vk*Vk)+(Ki*Vk)+(Kp));
Ql=Qnom *((Kz*Vk*Vk)+(Ki*Vk)+(Kp));
% Net Injected Curent.
% j=sqrt(-1);
Iinj = conj((Pl+j*Ql)/Vmeas);

== matlab function IEEE123bus_v2019b_Phasor_DPL_ZIPload/95 Y PQ/Embedded MATLAB Function ==
  data: Iinj output; Vmeas input; LoadType parameter; Vnom parameter; Pnom parameter; Qnom parameter; Vlim parameter
%Single Phase ZIP Load
%Author: Arun Suresh, University of North Carolina, Charlotte
%Iinj=((Pnom+jQnom)/Vmeas)'
function Iinj = InjectedCurrent(Vmeas,LoadType,Vnom,Pnom,Qnom,Vlim)
% Calculate Pl and Ql.
Kz=0;Ki=0;Kp=0;
Vk=(abs(Vmeas)/Vnom);%(Vmeas/Vnom)
switch LoadType  % 1 for Constant Z, 2 for Constant I and 3 for Constant P, 
    case 1
        Kz=1;
    case 2
        if Vk >= Vlim % convert to Constant Z load due to voltage violation
            Ki=1;
        else
            Kz=1;
        end
    case 3
        if Vk >= Vlim % convert to Constant Z load due to voltage violation
           Kp=1;
        else
            Kz=1;
        end          
 
end
Pl=Pnom *((Kz*Vk*Vk)+(Ki*Vk)+(Kp));
Ql=Qnom *((Kz*Vk*Vk)+(Ki*Vk)+(Kp));
% Net Injected Curent.
% j=sqrt(-1);
Iinj = conj((Pl+j*Ql)/Vmeas);

== matlab function IEEE123bus_v2019b_Phasor_DPL_ZIPload/28 Y I/Embedded MATLAB Function ==
  data: Iinj output; Vmeas input; LoadType parameter; Vnom parameter; Pnom parameter; Qnom parameter; Vlim parameter
%Single Phase ZIP Load
%Author: Arun Suresh, University of North Carolina, Charlotte
%Iinj=((Pnom+jQnom)/Vmeas)'
function Iinj = InjectedCurrent(Vmeas,LoadType,Vnom,Pnom,Qnom,Vlim)
% Calculate Pl and Ql.
Kz=0;Ki=0;Kp=0;
Vk=(abs(Vmeas)/Vnom);%(Vmeas/Vnom)
switch LoadType  % 1 for Constant Z, 2 for Constant I and 3 for Constant P, 
    case 1
        Kz=1;
    case 2
        if Vk >= Vlim % convert to Constant Z load due to voltage violation
            Ki=1;
        else
            Kz=1;
        end
    case 3
        if Vk >= Vlim % convert to Constant Z load due to voltage violation
           Kp=1;
        else
            Kz=1;
        end          
 
end
Pl=Pnom *((Kz*Vk*Vk)+(Ki*Vk)+(Kp));
Ql=Qnom *((Kz*Vk*Vk)+(Ki*Vk)+(Kp));
% Net Injected Curent.
% j=sqrt(-1);
Iinj = conj((Pl+j*Ql)/Vmeas);
